simulink model "long_quad"  (R2015a)
settings: Solver=ode45  StartTime=0.0  StopTime=20.0  RelTol=1e-3
values from neighbouring files (symbols this model uses):
  dm = 0.15    [init_quad.m]
  g = 9.81    [init_quad.m]
  J = 0.1    [init_quad.m]
  m = 1    [init_quad.m]
libraries: simulink_extras x1
settings Model: Creator=gislefh  LastModifiedBy=gislefh

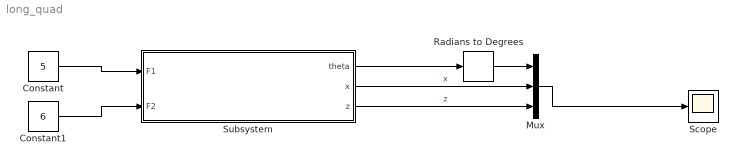
== system long_quad ==
  Constant : Constant  Value=5
  Constant1 : Constant  Value=6
  Mux : Mux  Inputs=3
  Radians to Degrees : simulink_extras/Transformations/Radians to Degrees
  Scope : Scope
      settings: ShowLegends=on
  Subsystem : Subsystem
  wires:
  Constant/1 -> Subsystem/1(F1)
  Constant1/1 -> Subsystem/2(F2)
  Mux/1 -> Scope/1
  Subsystem/2(x) -> Mux/2  "x"
  Subsystem/3("z ") -> Mux/3  "z"
  Subsystem/1(theta) -> Radians to Degrees/1
  Radians to Degrees/1 -> Mux/1

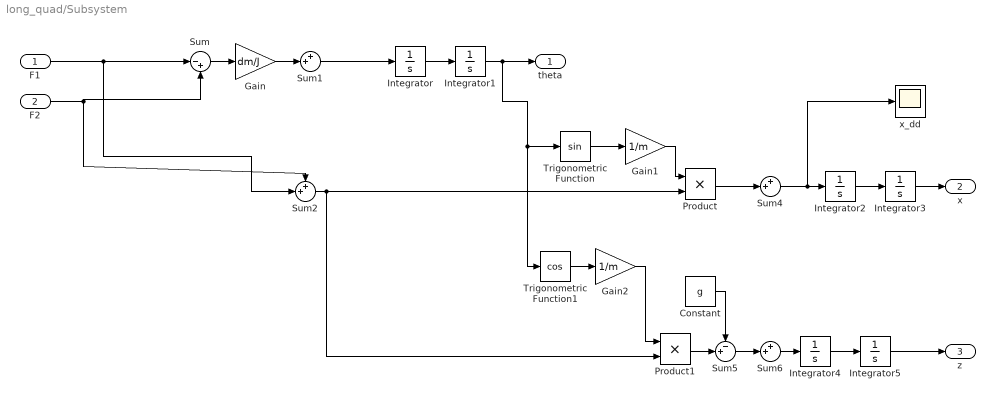
== system long_quad/Subsystem ==
  F1 : Inport
  F2 : Inport  Port=2
  Constant : Constant  Value=g
  Gain : Gain  Gain=dm/J
  Gain1 : Gain  Gain=1/m
  Gain2 : Gain  Gain=1/m
  Integrator{,1..5} (6 alike) : Integrator
  Product : Product
  Product1 : Product
  Sum : Sum  Inputs=|-+
  Sum{1..2,4,6} (4 alike) : Sum  Inputs=++|
  Sum5 : Sum  Inputs=-+|
  Trigonometric Function : Trigonometry
  Trigonometric Function1 : Trigonometry  Operator=cos
  x_dd : Scope
  theta : Outport
  x : Outport  Port=2
  "z " : Outport  Port=3
  wires:
  Integrator/1 -> Integrator1/1
  Integrator1/1 -> Trigonometric Function1/1, Trigonometric Function/1, theta/1
  F1/1 -> Sum2/2, Sum/1
  F2/1 -> Sum2/1, Sum/2
  Sum/1 -> Gain/1
  Gain/1 -> Sum1/2
  Sum1/1 -> Integrator/1
  Integrator2/1 -> Integrator3/1
  Integrator3/1 -> x/1
  Trigonometric Function/1 -> Gain1/1
  Gain1/1 -> Product/1
  Sum2/1 -> Product/2, Product1/2
  Constant/1 -> Sum5/1
  Product/1 -> Sum4/2
  Sum4/1 -> x_dd/1, Integrator2/1
  Integrator4/1 -> Integrator5/1
  Integrator5/1 -> "z "/1
  Gain2/1 -> Product1/1
  Product1/1 -> Sum5/2
  Sum5/1 -> Sum6/2
  Sum6/1 -> Integrator4/1
  Trigonometric Function1/1 -> Gain2/1
